simulink model "MetodoRele"  (R2025b)
(part 2 of 2)

  ZN-PID5 : slpidlib/PID Controller  Controller=PID  Form=Parallel  TimeDomain=Continuous-time  UseExternalTs=off  SampleTime=-1  IntegratorMethod=Forward Euler  FilterMethod=Forward Euler  ControllerParametersSource=internal  P=15.715  I=28.603  UseKiTs=off  D=2.1584  UseExternalDerivativeSource=off  N=100  UseFilter=on  TunerSelectOption=Transfer Function Based (PID Tuner App)  InitialConditionSource=internal  InitialConditionForIntegrator=0  InitialConditionForFilter=0  DifferentiatorICPrevScaledInput=0  ExternalReset=none  TrackingMode=off  Kt=1  LimitOutput=off  SatLimitsSource=internal  UpperSaturationLimit=inf  LowerSaturationLimit=-inf  LinearizeAsGain=on  AntiWindupMode=none  Kb=1  LimitIntegrator=off  UpperIntegratorSaturationLimit=inf  LowerIntegratorSaturationLimit=-inf  POutMin=[]  POutMax=[]  IOutMin=[]  IOutMax=[]  DOutMin=[]  DOutMax=[]  NOutMin=[]  NOutMax=[]  SumOutMin=[]  SumOutMax=[]  SaturationOutMin=[]  SaturationOutMax=[]  PParamMin=[]  PParamMax=[]  IParamMin=[]  IParamMax=[]  DParamMin=[]  DParamMax=[]  NParamMin=[]  NParamMax=[]  KbParamMin=[]  KbParamMax=[]  KtParamMin=[]  KtParamMax=[]  KbOutMin=[]  KbOutMax=[]  KtOutMin=[]  KtOutMax=[]  IntegratorOutMin=[]  IntegratorOutMax=[]  FilterOutMin=[]  FilterOutMax=[]  SumI1OutMin=[]  SumI1OutMax=[]  SumI2OutMin=[]  SumI2OutMax=[]  SumI3OutMin=[]  SumI3OutMax=[]  SumI4OutMin=[]  SumI4OutMax=[]  SumDOutMin=[]  SumDOutMax=[]  DifferentiatorOutMin=[]  DifferentiatorOutMax=[]  FilterDiffOutCoefMin=[]  FilterDiffOutCoefMax=[]  ReciprocalOutMin=[]  ReciprocalOutMax=[]  SumDenOutMin=[]  SumDenOutMax=[]  SumNumOutMin=[]  SumNumOutMax=[]  DivideOutMin=[]  DivideOutMax=[]  UdiffTsProdOutMin=[]  UdiffTsProdOutMax=[]  NTsProdOutMin=[]  NTsProdOutMax=[]  UintegralTsProdOutMin=[]  UintegralTsProdOutMax=[]  UngainTsProdOutMin=[]  UngainTsProdOutMax=[]  ClampingZeroOutDataTypeStr=Inherit: Inherit via back propagation  ClampingZeroOutMin=[]  ClampingZeroOutMax=[]  FilterDenConstantOutDataTypeStr=Inherit: Inherit via back propagation  FilterDenConstantOutMin=[]  FilterDenConstantOutMax=[]  PCopyOutDataTypeStr=Inherit: Inherit via back propagation  PCopyOutMin=[]  PCopyOutMax=[]  NCopyOutDataTypeStr=Inherit: Inherit via back propagation  NCopyOutMin=[]  NCopyOutMax=[]  IntegratorContinuousStateAttributes=''  IntegratorStateMustResolveToSignalObject=off  IntegratorRTWStateStorageClass=Auto  FilterContinuousStateAttributes=''  FilterStateMustResolveToSignalObject=off  FilterRTWStateStorageClass=Auto  ParallelPVariant=InternalParameters  IdealPVariant=Disabled  IVariant=InternalParameters  DVariant=InternalParameters  IntegratorVariant=Continuous  SatVariant=Disabled  AWVariant=Passthrough  PCopyVariant=Disabled  TRVariant=Disabled  FdbkBlocksVariant=Forward  IdealPFdbkVariant=Disabled  SatFdbkVariant=Disabled  DerivativeFilterVariant=ContFilter  NVariant=InternalParameters  NCopyVariant=Disabled  FilterICVariant=InternalICsFilter  IntegratorICVariant=InternalICs  ExternalResetVariant=Disabled  TRSumVariant=Passthrough  SumFdbkVariant=Disabled  SumVariant=Sum_PID  TsampFilterVariant=InternalTs  TsampNgainVariant=Passthrough  TsampIntegralVariant=Disabled_SignalSpec  ExternalSaturationOutDataTypeStr=Inherit: Same as second input  DerivativeSourceVariant=ErrorSignal  PreIntVariant=InternalPreInt
  ZN-PID6 : slpidlib/PID Controller  Controller=PID  Form=Parallel  TimeDomain=Continuous-time  UseExternalTs=off  SampleTime=-1  IntegratorMethod=Forward Euler  FilterMethod=Forward Euler  ControllerParametersSource=internal  P=12.98  I=17.231  UseKiTs=off  D=2.4445  UseExternalDerivativeSource=off  N=100  UseFilter=on  TunerSelectOption=Transfer Function Based (PID Tuner App)  InitialConditionSource=internal  InitialConditionForIntegrator=0  InitialConditionForFilter=0  DifferentiatorICPrevScaledInput=0  ExternalReset=none  TrackingMode=off  Kt=1  LimitOutput=off  SatLimitsSource=internal  UpperSaturationLimit=inf  LowerSaturationLimit=-inf  LinearizeAsGain=on  AntiWindupMode=none  Kb=1  LimitIntegrator=off  UpperIntegratorSaturationLimit=inf  LowerIntegratorSaturationLimit=-inf  POutMin=[]  POutMax=[]  IOutMin=[]  IOutMax=[]  DOutMin=[]  DOutMax=[]  NOutMin=[]  NOutMax=[]  SumOutMin=[]  SumOutMax=[]  SaturationOutMin=[]  SaturationOutMax=[]  PParamMin=[]  PParamMax=[]  IParamMin=[]  IParamMax=[]  DParamMin=[]  DParamMax=[]  NParamMin=[]  NParamMax=[]  KbParamMin=[]  KbParamMax=[]  KtParamMin=[]  KtParamMax=[]  KbOutMin=[]  KbOutMax=[]  KtOutMin=[]  KtOutMax=[]  IntegratorOutMin=[]  IntegratorOutMax=[]  FilterOutMin=[]  FilterOutMax=[]  SumI1OutMin=[]  SumI1OutMax=[]  SumI2OutMin=[]  SumI2OutMax=[]  SumI3OutMin=[]  SumI3OutMax=[]  SumI4OutMin=[]  SumI4OutMax=[]  SumDOutMin=[]  SumDOutMax=[]  DifferentiatorOutMin=[]  DifferentiatorOutMax=[]  FilterDiffOutCoefMin=[]  FilterDiffOutCoefMax=[]  ReciprocalOutMin=[]  ReciprocalOutMax=[]  SumDenOutMin=[]  SumDenOutMax=[]  SumNumOutMin=[]  SumNumOutMax=[]  DivideOutMin=[]  DivideOutMax=[]  UdiffTsProdOutMin=[]  UdiffTsProdOutMax=[]  NTsProdOutMin=[]  NTsProdOutMax=[]  UintegralTsProdOutMin=[]  UintegralTsProdOutMax=[]  UngainTsProdOutMin=[]  UngainTsProdOutMax=[]  ClampingZeroOutDataTypeStr=Inherit: Inherit via back propagation  ClampingZeroOutMin=[]  ClampingZeroOutMax=[]  FilterDenConstantOutDataTypeStr=Inherit: Inherit via back propagation  FilterDenConstantOutMin=[]  FilterDenConstantOutMax=[]  PCopyOutDataTypeStr=Inherit: Inherit via back propagation  PCopyOutMin=[]  PCopyOutMax=[]  NCopyOutDataTypeStr=Inherit: Inherit via back propagation  NCopyOutMin=[]  NCopyOutMax=[]  IntegratorContinuousStateAttributes=''  IntegratorStateMustResolveToSignalObject=off  IntegratorRTWStateStorageClass=Auto  FilterContinuousStateAttributes=''  FilterStateMustResolveToSignalObject=off  FilterRTWStateStorageClass=Auto  ParallelPVariant=InternalParameters  IdealPVariant=Disabled  IVariant=InternalParameters  DVariant=InternalParameters  IntegratorVariant=Continuous  SatVariant=Disabled  AWVariant=Passthrough  PCopyVariant=Disabled  TRVariant=Disabled  FdbkBlocksVariant=Forward  IdealPFdbkVariant=Disabled  SatFdbkVariant=Disabled  DerivativeFilterVariant=ContFilter  NVariant=InternalParameters  NCopyVariant=Disabled  FilterICVariant=InternalICsFilter  IntegratorICVariant=InternalICs  ExternalResetVariant=Disabled  TRSumVariant=Passthrough  SumFdbkVariant=Disabled  SumVariant=Sum_PID  TsampFilterVariant=InternalTs  TsampNgainVariant=Passthrough  TsampIntegralVariant=Disabled_SignalSpec  ExternalSaturationOutDataTypeStr=Inherit: Same as second input  DerivativeSourceVariant=ErrorSignal  PreIntVariant=InternalPreInt
  e=0.1 : Relay  OnSwitchValue=0.1  OffSwitchValue=-0.1  OnOutputValue=5  OffOutputValue=-5
  e=0.2 : Relay  OnSwitchValue=0.2  OffSwitchValue=-0.2  OnOutputValue=5  OffOutputValue=-5
  e=0.3 : Relay  OnSwitchValue=0.3  OffSwitchValue=-0.3  OnOutputValue=5  OffOutputValue=-5
  e=0.5 : Relay  OnSwitchValue=0.5  OffSwitchValue=-0.5  OnOutputValue=5  OffOutputValue=-5
  e=0.7 : Relay  OnSwitchValue=0.7  OffSwitchValue=-0.7  OnOutputValue=5  OffOutputValue=-5
  e=1 : Relay  OnSwitchValue=1  OffSwitchValue=-1  OnOutputValue=5  OffOutputValue=-5
  wires:
  TZN-PID6/1 -> Scope196/2, Scope200/3, Sum77/2
  Sum55/1 -> Tan-PID2/1
  Sum68/1 -> Corripio-PID4/1
  Sum64/1 -> ZN-PI4/1
  ZN-P4/1 -> Scope166/1, TZN-P4/1, Scope167/1
  Tan-PID5/1 -> Scope175/1, TTan-PID5/1, Scope176/1
  Sum73/1 -> Tan-PID5/1
  In20/1 -> Sum62/1, Scope161/7, Sum61/1, Sum60/1, Sum59/1, Sum58/1, Sum57/1
  ZN-P7e1/1 -> Scope205/1, TZN-P7e1/1, Scope206/1
  Sum56/1 -> Corripio-PID2/1
  Sum81/1 -> ZN-P7e1/1
  In23/1 -> Sum80/1, Scope200/7, Sum79/1, Sum78/1, Sum77/1, Sum76/1, Sum75/1
  Corripio-PID5/1 -> Scope177/1, TCorripio-PID5/1, Scope178/1
  TZN-P7e1/1 -> Scope205/2, Scope213/1, Sum81/2
  TZN-PID2/1 -> Scope144/2, Scope148/3, Sum53/2
  e=0.2/1 -> Scope83/1, Transfer Function1/1, Scope84/1
  Sum47/1 -> ZN-PID1/1
  TSmith-PID6/1 -> Scope198/2, Scope200/4, Sum78/2
  In18/1 -> Sum50/1, Scope135/7, Sum49/1, Sum48/1, Sum47/1, Sum46/1, Sum45/1
  Sum42/1 -> e=0.5/1
  In8/1 -> Sum44/1, Sum43/1, Sum42/1, Sum41/1, Sum40/1, Sum25/1
  ZN-P3/1 -> Scope153/1, TZN-P3/1, Scope154/1
  TSmith-PID1/1 -> Scope133/2, Scope135/4, Sum48/2
  TZN-P7e0,7/1 -> Scope207/2, Sum82/2, Scope213/2
  Sum66/1 -> Smith-PID4/1
  Sum57/1 -> ZN-P3/1
  e=0.3/1 -> Scope85/1, Transfer Function2/1, Scope86/1
  TTan-PID6/1 -> Scope188/2, Sum79/2, Scope200/5
  Transfer Function4/1 -> Scope119/2, Sum43/2
  Smith-PID1/1 -> Scope133/1, TSmith-PID1/1, Scope134/1
  TZN-PID7/1 -> Scope209/2, Scope213/3, Sum83/2
  Sum52/1 -> ZN-PI2/1
  TZN-PID1/1 -> Scope131/2, Scope135/3, Sum47/2
  ZN-PI4/1 -> Scope168/1, TZN-PI4/1, Scope169/1
  Corripio-PID1/1 -> Scope125/1, TCorripio-PID1/1, Scope126/1
  Tan-PID4/1 -> Scope162/1, TTan-PID4/1, Scope163/1
  e=0.7/1 -> Scope119/1, Transfer Function4/1, Scope120/1
  ZN-P5/1 -> Scope179/1, TZN-P5/1, Scope180/1
  Sum72/1 -> Smith-PID5/1
  TCorripio-PID6/1 -> Scope190/2, Scope200/6, Sum80/2
  Sum44/1 -> e=1/1
  Sum51/1 -> ZN-P2/1
  Sum48/1 -> Smith-PID1/1
  TZN-PID3/1 -> Scope157/2, Scope161/3, Sum59/2
  TSmith-PID2/1 -> Scope146/2, Scope148/4, Sum54/2
  Sum53/1 -> ZN-PID2/1
  Sum46/1 -> ZN-PI1/1
  ZN-PID6/1 -> Scope196/1, TZN-PID6/1, Scope197/1
  Sum69/1 -> ZN-P5/1
  TZN-P3/1 -> Scope153/2, Scope161/1, Sum57/2
  Sum71/1 -> ZN-PID5/1
  Sum58/1 -> ZN-PI3/1
  ZN-PI6/1 -> Scope194/1, TZN-PI6/1, Scope195/1
  Transfer Function3/1 -> Scope87/2, Sum42/2
  Sum60/1 -> Smith-PID3/1
  TZN-P4/1 -> Scope166/2, Scope174/1, Sum63/2
  Smith-PID4/1 -> Scope172/1, TSmith-PID4/1, Scope173/1
  Sum62/1 -> Corripio-PID3/1
  TZN-P1/1 -> Scope127/2, Scope135/1, Sum45/2
  e=0.5/1 -> Scope87/1, Transfer Function3/1, Scope88/1
  TZN-PID5/1 -> Scope183/2, Scope187/3, Sum71/2
  TTan-PID1/1 -> Scope123/2, Sum49/2, Scope135/5
  Sum45/1 -> ZN-P1/1
  ZN-PI1/1 -> Scope129/1, TZN-PI1/1, Scope130/1
  Sum76/1 -> ZN-PI6/1
  ZN-PID3/1 -> Scope157/1, TZN-PID3/1, Scope158/1
  Tan-PID3/1 -> Scope149/1, TTan-PID3/1, Scope150/1
  TSmith-PID4/1 -> Scope172/2, Scope174/4, Sum66/2
  Corripio-PID2/1 -> Scope138/1, TCorripio-PID2/1, Scope139/1
  In22/1 -> Sum74/1, Scope187/7, Sum73/1, Sum72/1, Sum71/1, Sum70/1, Sum69/1
  Sum61/1 -> Tan-PID3/1
  Sum75/1 -> ZN-P6/1
  TZN-P2/1 -> Scope140/2, Scope148/1, Sum51/2
  TCorripio-PID4/1 -> Scope164/2, Scope174/6, Sum68/2
  TZN-PI6/1 -> Scope194/2, Scope200/2, Sum76/2
  ZN-PID2/1 -> Scope144/1, TZN-PID2/1, Scope145/1
  Sum59/1 -> ZN-PID3/1
  ZN-PI2/1 -> Scope142/1, TZN-PI2/1, Scope143/1
  ZN-P6/1 -> Scope192/1, TZN-P6/1, Scope193/1
  ZN-P1/1 -> Scope127/1, TZN-P1/1, Scope128/1
  Sum82/1 -> ZN-P7e0.7/1
  TTan-PID3/1 -> Scope149/2, Sum61/2, Scope161/5
  Tan-PID1/1 -> Scope123/1, TTan-PID1/1, Scope124/1
  TZN-PI2/1 -> Scope142/2, Scope148/2, Sum52/2
  Sum70/1 -> ZN-PI5/1
  Sum63/1 -> ZN-P4/1
  TTan-PID4/1 -> Scope162/2, Sum67/2, Scope174/5
  Sum25/1 -> e=0.1/1
  TSmith-PID5/1 -> Scope185/2, Scope187/4, Sum72/2
  ZN-PID5/1 -> Scope183/1, TZN-PID5/1, Scope184/1
  Sum43/1 -> e=0.7/1
  Sum77/1 -> ZN-PID6/1
  Sum83/1 -> ZN-P7e0.5/1
  Sum67/1 -> Tan-PID4/1
  e=1/1 -> Scope121/1, Transfer Function5/1, Scope122/1
  ZN-P2/1 -> Scope140/1, TZN-P2/1, Scope141/1
  ZN-P7e0.5/1 -> Scope209/1, TZN-PID7/1, Scope210/1
  Sum80/1 -> Corripio-PID6/1
  TTan-PID2/1 -> Scope136/2, Sum55/2, Scope148/5
  Smith-PID3/1 -> Scope159/1, TSmith-PID3/1, Scope160/1
  Transfer Function1/1 -> Scope83/2, Sum40/2
  TCorripio-PID3/1 -> Scope151/2, Scope161/6, Sum62/2
  Sum40/1 -> e=0.2/1
  TCorripio-PID2/1 -> Scope138/2, Scope148/6, Sum56/2
  Transfer Function2/1 -> Scope85/2, Sum41/2
  In24/1 -> Sum83/1, Scope213/4, Sum82/1, Sum81/1
  ZN-PID1/1 -> Scope131/1, TZN-PID1/1, Scope132/1
  Tan-PID2/1 -> Scope136/1, TTan-PID2/1, Scope137/1
  Sum74/1 -> Corripio-PID5/1
  Transfer Function5/1 -> Scope121/2, Sum44/2
  TZN-PI4/1 -> Scope168/2, Scope174/2, Sum64/2
  TCorripio-PID5/1 -> Scope177/2, Scope187/6, Sum74/2
  Transfer Function/1 -> Scope81/2, Sum25/2
  Smith-PID6/1 -> Scope198/1, TSmith-PID6/1, Scope199/1
  Sum79/1 -> Tan-PID6/1
  Corripio-PID3/1 -> Scope151/1, TCorripio-PID3/1, Scope152/1
  Sum78/1 -> Smith-PID6/1
  Smith-PID5/1 -> Scope185/1, TSmith-PID5/1, Scope186/1
  TTan-PID5/1 -> Scope175/2, Sum73/2, Scope187/5
  TSmith-PID3/1 -> Scope159/2, Scope161/4, Sum60/2
  ZN-P7e0.7/1 -> Scope207/1, TZN-P7e0,7/1, Scope208/1
  TZN-PID4/1 -> Scope170/2, Scope174/3, Sum65/2
  Corripio-PID4/1 -> Scope164/1, TCorripio-PID4/1, Scope165/1
  Corripio-PID6/1 -> Scope190/1, TCorripio-PID6/1, Scope191/1
  ZN-PID4/1 -> Scope170/1, TZN-PID4/1, Scope171/1
  Tan-PID6/1 -> Scope188/1, TTan-PID6/1, Scope189/1
  e=0.1/1 -> Scope81/1, Transfer Function/1, Scope82/1
  In21/1 -> Sum68/1, Scope174/7, Sum67/1, Sum66/1, Sum65/1, Sum64/1, Sum63/1
  TZN-PI1/1 -> Scope129/2, Scope135/2, Sum46/2
  Sum65/1 -> ZN-PID4/1
  ZN-PI3/1 -> Scope155/1, TZN-PI3/1, Scope156/1
  In19/1 -> Sum56/1, Scope148/7, Sum55/1, Sum54/1, Sum53/1, Sum52/1, Sum51/1
  TZN-P6/1 -> Scope192/2, Scope200/1, Sum75/2
  TZN-P5/1 -> Scope179/2, Scope187/1, Sum69/2
  TCorripio-PID1/1 -> Scope125/2, Scope135/6, Sum50/2
  ZN-PI5/1 -> Scope181/1, TZN-PI5/1, Scope182/1
  TZN-PI3/1 -> Scope155/2, Scope161/2, Sum58/2
  Sum54/1 -> Smith-PID2/1
  Sum50/1 -> Corripio-PID1/1
  TZN-PI5/1 -> Scope181/2, Scope187/2, Sum70/2
  Smith-PID2/1 -> Scope146/1, TSmith-PID2/1, Scope147/1
  Sum49/1 -> Tan-PID1/1
  Sum41/1 -> e=0.3/1
